simulink model "model"  (R2015a)
settings: Solver=ode45  StartTime=0.0  StopTime=10.0  RelTol=1e-3
settings Model: Creator=Werner  LastModifiedBy=Werner

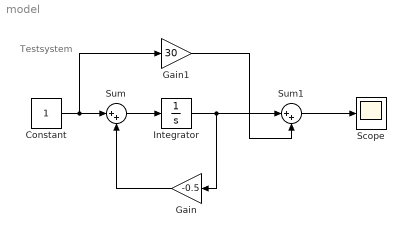
== system model ==
  note: Testsystem
  Constant : Constant
  Gain : Gain  Gain=-0.5
  Gain1 : Gain  Gain=30
  Integrator : Integrator
  Scope : Scope
  Sum : Sum  Inputs=|++
  Sum1 : Sum  Inputs=|++
  wires:
  Constant/1 -> Gain1/1, Sum/1
  Sum/1 -> Integrator/1
  Gain/1 -> Sum/2
  Integrator/1 -> Sum1/1, Gain/1
  Sum1/1 -> Scope/1
  Gain1/1 -> Sum1/2
